simulink model "adaptive_clean"  (Simulink 7.9)
settings: Solver=ode45  StartTime=0.0  StopTime=20  RelTol=1e-3
InitFcn:
  | startup_adaptive
values from neighbouring files (symbols this model uses):
  am = 5    [startup_adaptive.m]    (also in startup_exact.m)
  f1 = 5.0991    [startup_adaptive.m]    (also in startup_exact.m)
  f2 = 85.3455    [startup_adaptive.m]    (also in startup_exact.m)
  g1 = 13.8    [startup_adaptive.m]    (also in startup_exact.m)
  g2 = 41.1089    [startup_adaptive.m]    (also in startup_exact.m)
  gamma = 5000*[1 0 0 0 0 ... (first row only)    [startup_adaptive.m]
  kexact = -45.4545    [startup_adaptive.m]
  llim = -inf    [startup_adaptive.m]
  T = [1 2*zeta*wn wn^2]    [startup_adaptive.m]    (also in startup_exact.m)
  ulim = inf    [startup_adaptive.m]
libraries: simulink x2
settings Model: Creator=Prasad  LastModifiedBy=Narasimha Prasad
settings DebuggingCC: FcnCallInpInsideContextMsg=Use local settings
settings GRTTargetCC: CombineOutputUpdateFcns=off  GRTInterface=on

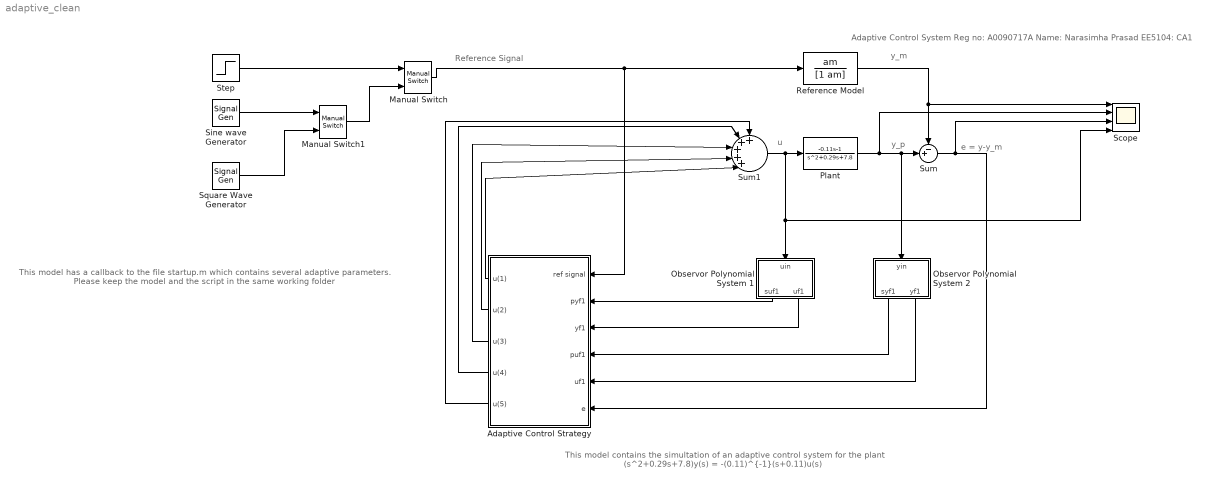
== system adaptive_clean ==
  note: Adaptive Control System
      | Reg no: A0090717A
      | Name: Narasimha Prasad
      | EE5104: CA1
  note: This model contains the simultation of an adaptive control system for the plant (s^2+0.29s+7.8)y(s) = -(0.11)^{-1}(s+0.11)u(s)
  note: This model has a callback
      | to the file startup.m which
      | contains several adaptive
      | parameters. Please keep
      |  the model and the script
      | in the same working folder
  note: Reference Signal
  note: u
  note: y_p
  note: y_m
  note: e = y-y_m
  Adaptive Control Strategy : Subsystem
  Manual Switch : simulink/Signal Routing/Manual Switch  sw=0  action=0  varsize=off
  Manual Switch1 : simulink/Signal Routing/Manual Switch  sw=1  action=0  varsize=off
  Observor Polynomial System 1 : Subsystem
  Observor Polynomial System 2 : Subsystem
  Plant : TransferFcn  Numerator=[-0.11 -1]  Denominator=[1 0.29 7.8]
  Reference Model : TransferFcn  Numerator=am  Denominator=[1 am]
  Scope : Scope  NumInputPorts=4
      settings: TimeRange=8  YMin=-2~-20~-0.1~-500  YMax=2~20~0.1~1000
  Sine wave Generator : SignalGenerator  Amplitude=10  Frequency=2  Units=rad/sec
  Square Wave Generator : SignalGenerator  WaveForm=square  Frequency=2.2  Units=rad/sec
  Step : Step  SampleTime=0
  Sum : Sum  Inputs=-+|
  Sum1 : Sum  Inputs=+++++|
  wires:
  Reference Model/1 -> Sum/1, Scope/1
  Plant/1 -> Sum/2, Observor Polynomial System 2/1(yin), Scope/2
  Sum1/1 -> Plant/1, Observor Polynomial System 1/1(uin), Scope/4
  Sum/1 -> Adaptive Control Strategy/6(e), Scope/3
  Manual Switch/1 -> Reference Model/1, Adaptive Control Strategy/1(ref signal)
  Sine wave Generator/1 -> Manual Switch1/1
  Square Wave Generator/1 -> Manual Switch1/2
  Step/1 -> Manual Switch/1
  Manual Switch1/1 -> Manual Switch/2
  Observor Polynomial System 1/1(suf1) -> Adaptive Control Strategy/2(pyf1)
  Observor Polynomial System 1/2(uf1) -> Adaptive Control Strategy/3(yf1)
  Observor Polynomial System 2/1(syf1) -> Adaptive Control Strategy/4(puf1)
  Observor Polynomial System 2/2(yf1) -> Adaptive Control Strategy/5(uf1)
  Adaptive Control Strategy/1(u(1)) -> Sum1/5
  Adaptive Control Strategy/2(u(2)) -> Sum1/4
  Adaptive Control Strategy/3(u(3)) -> Sum1/3
  Adaptive Control Strategy/4(u(4)) -> Sum1/2
  Adaptive Control Strategy/5(u(5)) -> Sum1/1

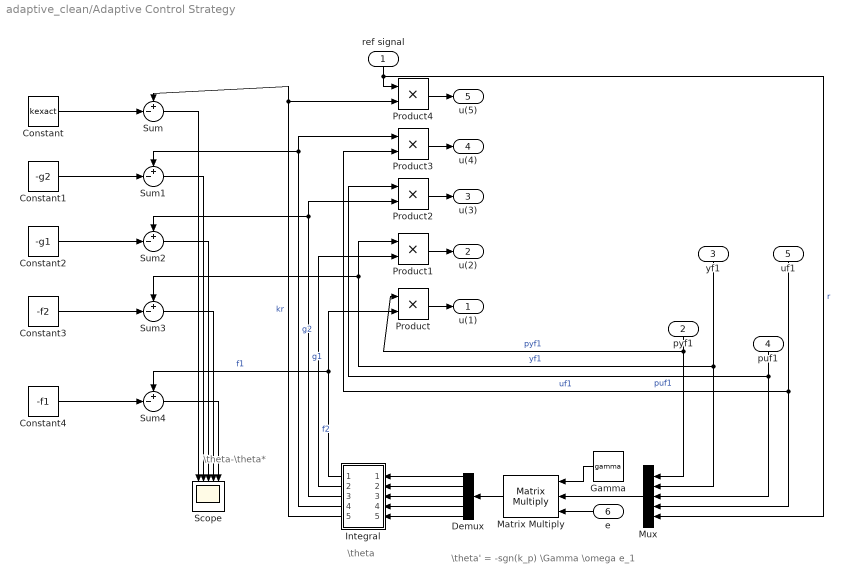
== system adaptive_clean/Adaptive Control Strategy ==
  note: \theta' = -sgn(k_p) \Gamma \omega e_1
  note: \theta
  note: \theta-\theta*
  ref signal : Inport
  pyf1 : Inport  Port=2
  yf1 : Inport  Port=3
  puf1 : Inport  Port=4
  uf1 : Inport  Port=5
  e : Inport  Port=6
  Constant : Constant  Value=kexact
  Constant1 : Constant  Value=-g2
  Constant2 : Constant  Value=-g1
  Constant3 : Constant  Value=-f2
  Constant4 : Constant  Value=-f1
  Demux : Demux  Outputs=5
  Gamma : Constant  Value=gamma  VectorParams1D=off
  Integral : Subsystem
  Matrix Multiply : Product  Inputs=3  Multiplication=Matrix(*)
  Mux : Mux  Inputs=5
  Product{,1..4} (5 alike) : Product  RndMeth=Zero
  Scope : Scope  NumInputPorts=5
      settings: TimeRange=20  YMin=-20~40~-20~40~-100  YMax=20~55~40~120~50
  Sum{,1..4} (5 alike) : Sum  Inputs=+-|
  u(1) : Outport
  u(2) : Outport  Port=2
  u(3) : Outport  Port=3
  u(4) : Outport  Port=4
  u(5) : Outport  Port=5
  wires:
  Integral/5(Out5) -> Product4/2, Sum/1  "kr"
  Demux/3 -> Integral/3(In3)
  Demux/5 -> Integral/5(In5)
  Demux/4 -> Integral/4(In4)
  Demux/2 -> Integral/2(In2)
  Demux/1 -> Integral/1(In1)
  Matrix Multiply/1 -> Demux/1
  Mux/1 -> Matrix Multiply/2
  uf1/1 -> Mux/4, Product3/2  "uf1"
  puf1/1 -> Mux/3, Product2/1  "puf1"
  yf1/1 -> Mux/2, Product1/1, Sum3/1  "yf1"
  pyf1/1 -> Mux/1, Product/1  "pyf1"
  ref signal/1 -> Mux/5, Product4/1  "r"
  Product4/1 -> u(5)/1
  Product3/1 -> u(4)/1
  Product2/1 -> u(3)/1
  Product1/1 -> u(2)/1
  Product/1 -> u(1)/1
  e/1 -> Matrix Multiply/3
  Integral/4(Out4) -> Product3/1, Sum1/1  "g2"
  Integral/3(Out3) -> Product2/2, Sum2/1  "g1"
  Integral/2(Out2) -> Product1/2  "f2"
  Integral/1(Out1) -> Product/2, Sum4/1  "f1"
  Gamma/1 -> Matrix Multiply/1
  Constant/1 -> Sum/2
  Constant1/1 -> Sum1/2
  Constant2/1 -> Sum2/2
  Constant3/1 -> Sum3/2
  Constant4/1 -> Sum4/2
  Sum/1 -> Scope/1
  Sum1/1 -> Scope/2
  Sum2/1 -> Scope/3
  Sum3/1 -> Scope/4
  Sum4/1 -> Scope/5

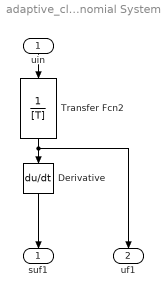
== system adaptive_clean/Observor Polynomial System 1 ==
  uin : Inport
  Derivative : Derivative
  Transfer Fcn2 : TransferFcn  Denominator=[T]
  suf1 : Outport
  uf1 : Outport  Port=2
  wires:
  Transfer Fcn2/1 -> uf1/1, Derivative/1
  uin/1 -> Transfer Fcn2/1
  Derivative/1 -> suf1/1

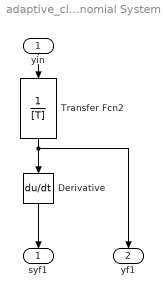
== system adaptive_clean/Observor Polynomial System 2 ==
  yin : Inport
  Derivative : Derivative
  Transfer Fcn2 : TransferFcn  Denominator=[T]
  syf1 : Outport
  yf1 : Outport  Port=2
  wires:
  Transfer Fcn2/1 -> yf1/1, Derivative/1
  yin/1 -> Transfer Fcn2/1
  Derivative/1 -> syf1/1

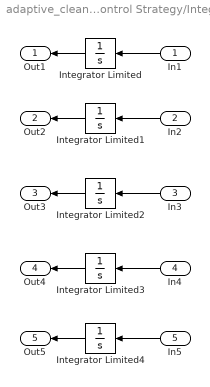
== system adaptive_clean/Adaptive Control Strategy/Integral ==
  In1 : Inport
  In2 : Inport  Port=2
  In3 : Inport  Port=3
  In4 : Inport  Port=4
  In5 : Inport  Port=5
  Integrator Limited{,1..4} (5 alike) : Integrator  LimitOutput=on  UpperSaturationLimit=ulim  LowerSaturationLimit=llim
  Out1 : Outport
  Out2 : Outport  Port=2
  Out3 : Outport  Port=3
  Out4 : Outport  Port=4
  Out5 : Outport  Port=5
  wires:
  In1/1 -> Integrator Limited/1
  Integrator Limited/1 -> Out1/1
  In2/1 -> Integrator Limited1/1
  Integrator Limited1/1 -> Out2/1
  In3/1 -> Integrator Limited2/1
  Integrator Limited2/1 -> Out3/1
  In4/1 -> Integrator Limited3/1
  Integrator Limited3/1 -> Out4/1
  In5/1 -> Integrator Limited4/1
  Integrator Limited4/1 -> Out5/1
